simulink model "trajectory"  (R2017b)
settings: Solver=ode4  StartTime=0.0  StopTime=T  FixedStep=dt  RelTol=1e-3
values from neighbouring files (symbols this model uses):
  acc_noise = (0.11/sqrt(3600))^2 *1    [gene_traj.m]
  gyro_noise = (0.66/sqrt(3600)/180*pi)^2 *1    [gene_traj.m]
undefined symbols (not defined in the file or in its folder): att0, Earth, WGS84
libraries: aerolibconvert2 x2, aerolibgravity2 x2, aerolibutil x2, sharedtransform x2, aerolib6dof2 x1, aerolibnav x1, simulink x1
settings Model: Creator=longteng  LastModifiedBy=longt
settings Model: ModifiedComment=|
  | longt -- Wed Mar 07 22:17:09 2018 -- Version 1.5
  | Modify Wb and Fb line.
settings Model: ModifiedHistory=|
  | longt -- Wed Mar 07 22:17:09 2018 -- Version 1.5
  | Modify Wb and Fb line.
  | 
  | longt -- Tue Feb 06 13:44:48 2018 -- Version 1.4
  | delete imu quantize
  | 
  | longteng -- Fri Jan 26 13:47:11 2018 -- Version 1.3
  | modify trajectory.slx to be compatible with low vrsion
  | 
  | longteng -- Thu Jan 11 22:14:16 2018 -- Version 1.2
  | Disable tout output.
  | 
  | longteng -- Thu Jan 11 21:47:38 2018 -- Version 1.1
  | Create model.
  | Tracking the target trajectory through the control system, and outputing acceleration and angular velocity.
settings DataIOCC: SaveOutput=off  SignalLogging=off  DSMLogging=off  SaveTime=off

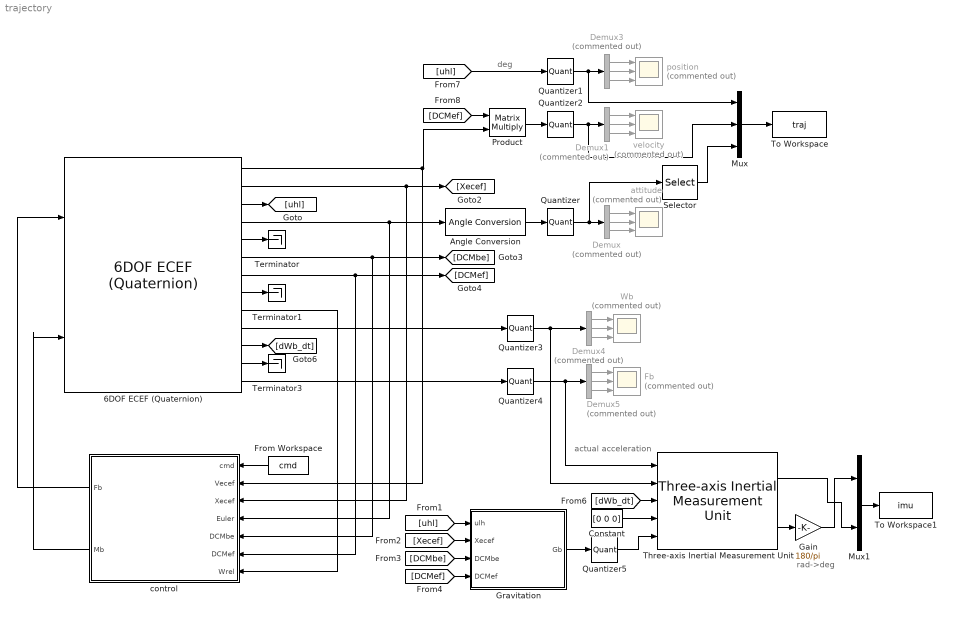
== system trajectory ==
  note: rad->deg
  note: actual acceleration
  note: deg
  6DOF ECEF (Quaternion) : aerolib6dof2/6DOF ECEF (Quaternion)  units=Metric (MKS)  mtype=Fixed  xg_0=p0  Vm_0=vb0  eul_0=[att0(3) att0(2) att0(1)]/180*pi  pm_0=[0 0 0]  mass_0=1.0  mass_e=0.5  mass_f=2.0  inertia=eye(3)  inertia_e=eye(3)  inertia_f=2*eye(3)  vre_flag=on  abi_flag=on  ptype=Earth (WGS84)  R=6378137  F=1/298.257223563  w_E=7292115e-11  angle_in=Internal  LG0=0
      settings: SourceProductName=Aerospace Blockset  SourceProductBaseCode=AE
  Angle Conversion : aerolibconvert2/Angle Conversion  IU=rad  OU=deg
  Constant : Constant  Value=[0 0 0]
  Demux{,1,3..5} (5 alike) : Demux  Commented=on  Outputs=3
  Fb : Scope  Commented=on  NumInputPorts=3
  From Workspace : FromWorkspace  VariableName=cmd  SampleTime=0  OutputAfterFinalValue=Setting to zero
  Gain : Gain  Gain=180/pi
  Gravitation : Subsystem
  Mux : Mux  Inputs=3
  Mux1 : Mux  Inputs=2
  Product : Product  Multiplication=Matrix(*)
  Quantizer : Quantizer  QuantizationInterval=1e-4
  Quantizer1 : Quantizer  QuantizationInterval=[1e-10 1e-10 0.001]
  Quantizer2 : Quantizer  QuantizationInterval=0.001
  Quantizer3 : Quantizer  QuantizationInterval=1e-12
  Quantizer4 : Quantizer  QuantizationInterval=1e-12
  Quantizer5 : Quantizer  QuantizationInterval=1e-12
  Selector : Selector  InputPortWidth=3  IndexOptions=Index vector (dialog)  Indices=[3 2 1]  OutputSizes=1
  Terminator : Terminator
  Terminator1 : Terminator
  Terminator3 : Terminator
  Three-axis Inertial Measurement Unit : aerolibnav/Three-axis Inertial Measurement Unit  units=Metric (MKS)  imu=[0 0 0]  i_Ts=dt  dtype_a=off  w_a=190  z_a=0.707  a_sf_cc=[1 0 0; 0 1 0; 0 0 1]  a_bias=acc_bias  a_sat="[-inf  -inf  -inf  inf inf inf]"  dtype_g=off  w_g=190  z_g=0.707  g_sf_cc=[1 0 0; 0 1 0; 0 0 1]  g_bias=gyro_bias  g_sens=[0 0 0]  g_sat="[-inf  -inf  -inf  inf inf inf]"  i_rand=on  i_seeds=noise_seeds  i_pow=[acc_noise*ones(1,3),gyro_noise*ones(1,3)]
  To Workspace : ToWorkspace  VariableName=traj  SampleTime=-1
  To Workspace1 : ToWorkspace  VariableName=imu  SampleTime=-1
  Wb : Scope  Commented=on  NumInputPorts=3
  attitude : Scope  Commented=on  NumInputPorts=3
  control : Subsystem
  position : Scope  Commented=on  NumInputPorts=3
  velocity : Scope  Commented=on  NumInputPorts=3
  wires:
  Demux/1 -> attitude/1
  Demux/2 -> attitude/2
  Demux/3 -> attitude/3
  Demux3/1 -> position/1
  Demux3/2 -> position/2
  Demux3/3 -> position/3
  From Workspace/1 -> control/1(cmd)
  6DOF ECEF (Quaternion)/1 -> Product/2, control/2(Vecef)
  6DOF ECEF (Quaternion)/2 -> [Xecef], control/3(Xecef)
  6DOF ECEF (Quaternion)/4 -> Angle Conversion/1, control/4(Euler)
  6DOF ECEF (Quaternion)/6 -> [DCMbe], control/5(DCMbe)
  6DOF ECEF (Quaternion)/7 -> [DCMef], control/6(DCMef)
  control/1(Fb) -> 6DOF ECEF (Quaternion)/1
  Angle Conversion/1 -> Quantizer/1
  6DOF ECEF (Quaternion)/3 -> [uhl]
  Demux1/3 -> velocity/3
  Demux1/2 -> velocity/2
  Demux1/1 -> velocity/1
  Product/1 -> Quantizer2/1
  control/2(Mb) -> 6DOF ECEF (Quaternion)/2
  6DOF ECEF (Quaternion)/9 -> control/7(Wrel)
  Quantizer/1 -> Selector/1, Demux/1
  Quantizer1/1 -> Mux/1, Demux3/1
  Quantizer2/1 -> Mux/2, Demux1/1
  6DOF ECEF (Quaternion)/10 -> Quantizer3/1
  Demux4/1 -> Wb/1
  Demux4/2 -> Wb/2
  Demux4/3 -> Wb/3
  Demux5/1 -> Fb/1
  Demux5/2 -> Fb/2
  Demux5/3 -> Fb/3
  6DOF ECEF (Quaternion)/5 -> Terminator/1
  6DOF ECEF (Quaternion)/8 -> Terminator1/1
  6DOF ECEF (Quaternion)/12 -> Terminator3/1
  Mux/1 -> To Workspace/1
  Quantizer3/1 -> Three-axis Inertial Measurement Unit/2, Demux4/1
  [DCMbe] -> Gravitation/3(DCMbe)
  [uhl] -> Gravitation/1(ulh)
  [Xecef] -> Gravitation/2(Xecef)
  [DCMef] -> Gravitation/4(DCMef)
  Gravitation/1(Gb) -> Quantizer5/1
  Constant/1 -> Three-axis Inertial Measurement Unit/4
  6DOF ECEF (Quaternion)/11 -> [dWb_dt]
  [dWb_dt] -> Three-axis Inertial Measurement Unit/3
  Quantizer4/1 -> Three-axis Inertial Measurement Unit/1, Demux5/1
  Selector/1 -> Mux/3
  [uhl] -> Quantizer1/1
  [DCMef] -> Product/1
  Quantizer5/1 -> Three-axis Inertial Measurement Unit/5
  Mux1/1 -> To Workspace1/1
  Three-axis Inertial Measurement Unit/2 -> Gain/1
  Gain/1 -> Mux1/1
  Three-axis Inertial Measurement Unit/1 -> Mux1/2
  6DOF ECEF (Quaternion)/13 -> Quantizer4/1

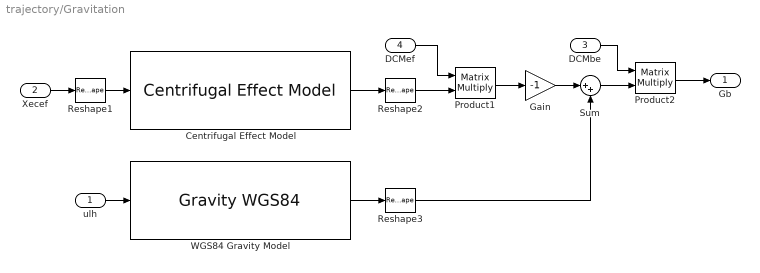
== system trajectory/Gravitation ==
  ulh : Inport
  Xecef : Inport  Port=2
  DCMbe : Inport  Port=3
  DCMef : Inport  Port=4
  Centrifugal Effect Model : aerolibgravity2/Centrifugal Effect Model  ptype=Earth  omega=7.2921150e-05  rate_loc=off
      settings: SourceProductName=Aerospace Blockset  SourceProductBaseCode=AE
  Gain : Gain  Gain=-1
  Product1 : Product  Multiplication=Matrix(*)
  Product2 : Product  Multiplication=Matrix(*)
  Reshape1 : Reshape
  Reshape2 : Reshape
  Reshape3 : Reshape
  Sum : Sum  Inputs=|++
  "WGS84 Gravity Model  " : GravityWGS84
  Gb : Outport
  wires:
  "WGS84 Gravity Model  "/1 -> Reshape3/1
  Product2/1 -> Gb/1
  Reshape1/1 -> Centrifugal Effect Model/1
  Reshape2/1 -> Product1/2
  Centrifugal Effect Model/1 -> Reshape2/1
  ulh/1 -> "WGS84 Gravity Model  "/1
  DCMbe/1 -> Product2/1
  Xecef/1 -> Reshape1/1
  DCMef/1 -> Product1/1
  Product1/1 -> Gain/1
  Sum/1 -> Product2/2
  Gain/1 -> Sum/1
  Reshape3/1 -> Sum/2

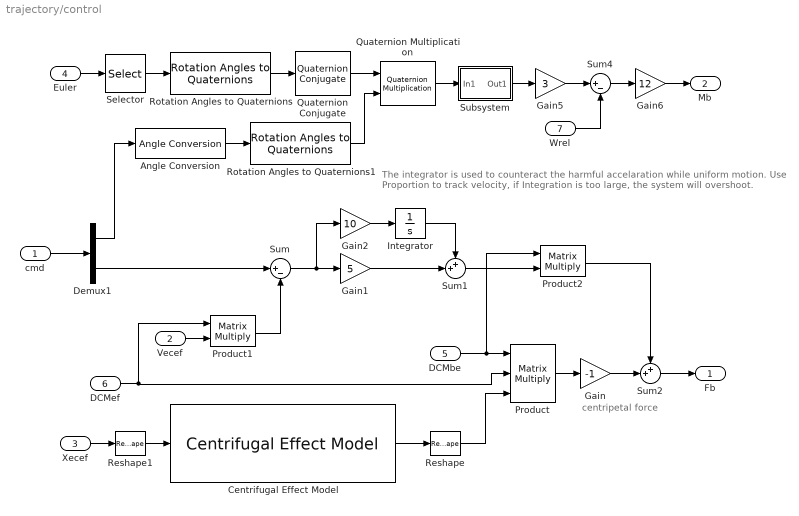
== system trajectory/control ==
  note: The integrator is used to counteract the harmful accelaration while uniform motion.
      | Use Proportion to track velocity, if Integration is too large, the system will overshoot.
  note: centripetal force
  cmd : Inport
  Vecef : Inport  Port=2
  Xecef : Inport  Port=3
  Euler : Inport  Port=4
  DCMbe : Inport  Port=5
  DCMef : Inport  Port=6
  Wrel : Inport  Port=7
  Angle Conversion : aerolibconvert2/Angle Conversion  IU=deg  OU=rad
  Centrifugal Effect Model : aerolibgravity2/Centrifugal Effect Model  ptype=Earth  omega=7.2921150e-05  rate_loc=off
      settings: SourceProductName=Aerospace Blockset  SourceProductBaseCode=AE
  Demux1 : Demux  Outputs=[3 3]
  Gain : Gain  Gain=-1
  Gain1 : Gain  Gain=5
  Gain2 : Gain  Gain=10
  Gain5 : Gain  Gain=3
  Gain6 : Gain  Gain=12
  Integrator : Integrator  LimitOutput=on  UpperSaturationLimit=0.2  LowerSaturationLimit=-0.2
  Product : Product  Inputs=3  Multiplication=Matrix(*)
  Product1 : Product  Multiplication=Matrix(*)
  Product2 : Product  Multiplication=Matrix(*)
  Quaternion Conjugate : aerolibutil/Quaternion Conjugate
      settings: SourceProductName=Aerospace Blockset  SourceProductBaseCode=AE
  Quaternion Multiplication : aerolibutil/Quaternion Multiplication
  Reshape : Reshape
  Reshape1 : Reshape
  Rotation Angles to Quaternions : sharedtransform/Rotation Angles to Quaternions  rotationOrder=ZYX
      settings: SourceProductName=Aerospace Blockset  SourceProductBaseCode=AE
  Rotation Angles to Quaternions1 : sharedtransform/Rotation Angles to Quaternions  rotationOrder=ZYX
      settings: SourceProductName=Aerospace Blockset  SourceProductBaseCode=AE
  Selector : Selector  InputPortWidth=3  IndexOptions=Index vector (dialog)  Indices=[3 2 1]  OutputSizes=1
  Subsystem : Subsystem
  Sum : Sum  Inputs=|+-
  Sum1 : Sum  Inputs=++|
  Sum2 : Sum  Inputs=++|
  Sum4 : Sum  Inputs=|+-
  Fb : Outport
  Mb : Outport  Port=2
  wires:
  Sum2/1 -> Fb/1
  Product1/1 -> Sum/2
  Gain2/1 -> Integrator/1
  Product2/1 -> Sum2/1
  Gain/1 -> Sum2/2
  Sum/1 -> Gain2/1, Gain1/1
  Vecef/1 -> Product1/2
  Centrifugal Effect Model/1 -> Reshape/1
  DCMbe/1 -> Product2/1, Product/1
  Reshape/1 -> Product/3
  cmd/1 -> Demux1/1
  Integrator/1 -> Sum1/1
  Demux1/2 -> Sum/1
  Gain1/1 -> Sum1/2
  Xecef/1 -> Reshape1/1
  Product/1 -> Gain/1
  DCMef/1 -> Product1/1, Product/2
  Reshape1/1 -> Centrifugal Effect Model/1
  Wrel/1 -> Sum4/2
  Sum4/1 -> Gain6/1
  Gain6/1 -> Mb/1
  Sum1/1 -> Product2/2
  Euler/1 -> Selector/1
  Demux1/1 -> Angle Conversion/1
  Selector/1 -> Rotation Angles to Quaternions/1
  Angle Conversion/1 -> Rotation Angles to Quaternions1/1
  Rotation Angles to Quaternions/1 -> Quaternion Conjugate/1
  Rotation Angles to Quaternions1/1 -> Quaternion Multiplication/2
  Quaternion Conjugate/1 -> Quaternion Multiplication/1
  Gain5/1 -> Sum4/1
  Quaternion Multiplication/1 -> Subsystem/1(In1)
  Subsystem/1(Out1) -> Gain5/1

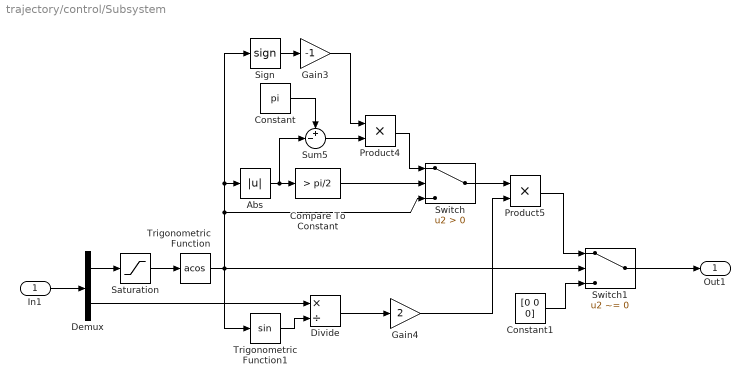
== system trajectory/control/Subsystem ==
  In1 : Inport
  Abs : Abs
  Compare To Constant : simulink/Logic and Bit Operations/Compare To Constant  relop=>  const=pi/2  OutDataTypeStr=boolean
  Constant : Constant  Value=pi
  Constant1 : Constant  Value=[0 0 0]
  Demux : Demux  Outputs=[1 3]
  Divide : Product  Inputs=*/
  Gain3 : Gain  Gain=-1
  Gain4 : Gain  Gain=2
  Product4 : Product
  Product5 : Product
  Saturation : Saturate  UpperLimit=1  LowerLimit=-1
  Sign : Signum
  Sum5 : Sum  Inputs=+-|
  Switch : Switch  Criteria=u2 > Threshold
  Switch1 : Switch  Criteria=u2 ~= 0
  Trigonometric Function : Trigonometry  Operator=acos
  Trigonometric Function1 : Trigonometry
  Out1 : Outport
  wires:
  Demux/1 -> Saturation/1
  In1/1 -> Demux/1
  Gain3/1 -> Product4/1
  Constant/1 -> Sum5/1
  Trigonometric Function/1 -> Trigonometric Function1/1, Switch1/2, Sign/1, Abs/1, Switch/3
  Abs/1 -> Sum5/2, Compare To Constant/1
  Constant1/1 -> Switch1/3
  Switch1/1 -> Out1/1
  Switch/1 -> Product5/1
  Gain4/1 -> Product5/2
  Trigonometric Function1/1 -> Divide/2
  Demux/2 -> Divide/1
  Divide/1 -> Gain4/1
  Product5/1 -> Switch1/1
  Sign/1 -> Gain3/1
  Compare To Constant/1 -> Switch/2
  Product4/1 -> Switch/1
  Sum5/1 -> Product4/2
  Saturation/1 -> Trigonometric Function/1
